simulink model "Utkarsh_2005574_W3_P3"  (R2020b)
settings: Solver=ode45  StartTime=0.0  StopTime=25  MaxStep=0.01  RelTol=1e-3  AbsTol=1e-6
PostLoadFcn:
  | g = 32.18;
  | v0 = 88;
  | Rr = 15/12;
  | Kf = 1;
  | m = 50;
  | PBmax = 1500;
  | TB = 0.01;
  | I = 5;
  | 
  | slip = (0:.05:1.0);
  | mu = [0 .4 .8 .97 1.0 .98 .96 .94 .92 .9 .88 .855 .83 .81 .79 .77 .75 .73 .72 .71 .7];
  | ctrl = 1;
InitFcn:
  | g = 32.18;
  | v0 = 88;
  | Rr = 15/12;
  | Kf = 1;
  | m = 50;
  | PBmax = 1500;
  | TB = 0.01;
  | I = 5;
  | 
  | slip = (0:.05:1.0);
  | mu = [0 .4 .8 .97 1.0 .98 .96 .94 .92 .9 .88 .855 .83 .81 .79 .77 .75 .73 .72 .71 .7];
  | ctrl = 1;
settings Model: Creator=home  LastModifiedBy=home

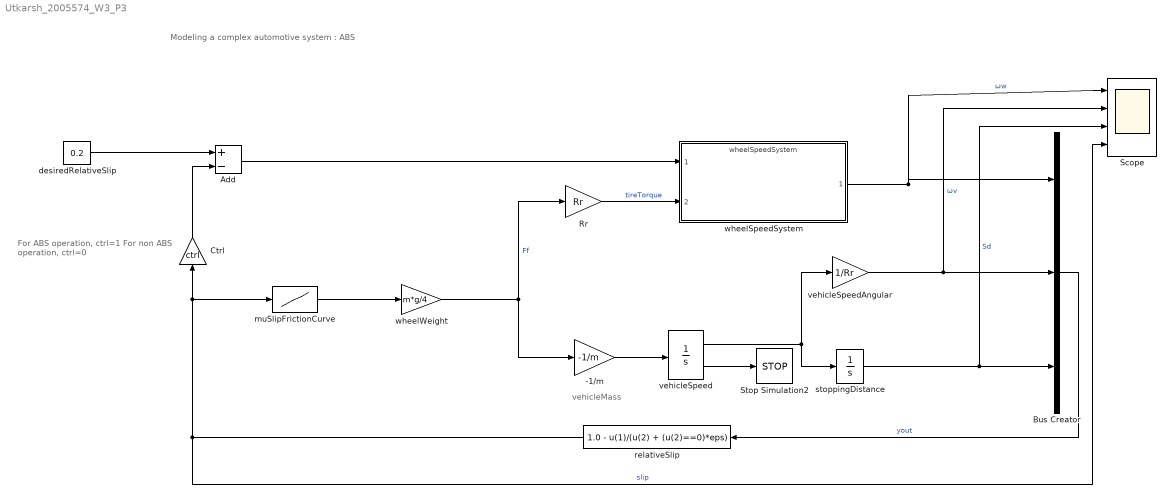
== system Utkarsh_2005574_W3_P3 ==
  note: vehicleMass
  note: For ABS operation,
      | ctrl=1
      | For non ABS operation,
      | ctrl=0
  note: Modeling a complex automotive system : ABS
  -1/m : Gain  Gain=-1/m  SaturateOnIntegerOverflow=on  OutDataTypeStr=Inherit: Same as input  ParamDataTypeStr=Inherit: Same as input
  Add : Sum  Inputs=+-
  Bus Creator : BusCreator  Inputs=3
  Ctrl : Gain  Gain=ctrl  SaturateOnIntegerOverflow=on  OutDataTypeStr=Inherit: Same as input  ParamDataTypeStr=Inherit: Same as input
  Rr : Gain  Gain=Rr  SaturateOnIntegerOverflow=on  OutDataTypeStr=Inherit: Same as input  ParamDataTypeStr=Inherit: Same as input
  Scope : Scope  NumInputPorts=4
  Stop Simulation2 : Stop
  desiredRelativeSlip : Constant  Value=0.2
  muSlipFrictionCurve : Lookup_n-D  NumberOfTableDimensions=1  BreakpointsForDimension1=slip  Table=mu  SaturateOnIntegerOverflow=on  InputSameDT=on
  relativeSlip : Fcn  Expr=1.0 - u(1)/(u(2) + (u(2)==0)*eps)
  stoppingDistance : Integrator  UpperSaturationLimit=1000  LowerSaturationLimit=0
  vehicleSpeed : Integrator  InitialCondition=v0  LimitOutput=on  UpperSaturationLimit=1000  LowerSaturationLimit=0  ShowSaturationPort=on
  vehicleSpeedAngular : Gain  Gain=1/Rr  SaturateOnIntegerOverflow=on  OutDataTypeStr=Inherit: Same as input  ParamDataTypeStr=Inherit: Same as input
  wheelSpeedSystem : ModelReference  ModelNameDialog=wheelSpeedSystem  SimulationMode=Normal  ModelReferenceVersion=1.16
  wheelWeight : Gain  Gain=m*g/4  SaturateOnIntegerOverflow=on  OutDataTypeStr=Inherit: Same as input  ParamDataTypeStr=Inherit: Same as input
  wires:
  Add/1 -> wheelSpeedSystem/1
  muSlipFrictionCurve/1 -> wheelWeight/1
  Rr/1 -> wheelSpeedSystem/2  "tireTorque"
  desiredRelativeSlip/1 -> Add/1
  vehicleSpeedAngular/1 -> Scope/2, Bus Creator/2  "ωv"
  -1/m/1 -> vehicleSpeed/1
  relativeSlip/1 -> muSlipFrictionCurve/1, Ctrl/1, Scope/4  "slip"
  Ctrl/1 -> Add/2
  vehicleSpeed/2 -> Stop Simulation2/1
  Bus Creator/1 -> relativeSlip/1  "yout"
  stoppingDistance/1 -> Bus Creator/3, Scope/3  "Sd"
  wheelWeight/1 -> -1/m/1, Rr/1  "Ff"
  vehicleSpeed/1 -> vehicleSpeedAngular/1, stoppingDistance/1
  wheelSpeedSystem/1 -> Bus Creator/1, Scope/1  "ωw"
